simulink model "prob3"  (R2020b)
settings: Solver=VariableStepAuto  StartTime=0.0  StopTime=10.0  RelTol=1e-3
model workspace: external: MATLAB File C:\Users\deves\MATLAB\Projects\W2_problem3\data3.m (data not in the file)
values from neighbouring files (symbols this model uses):
  b = 50    [data3.m]
  M = 1000    [data3.m]
  U = 500    [data3.m]
settings Model: OrderedModelArguments=off  Creator=deves  LastModifiedBy=deves

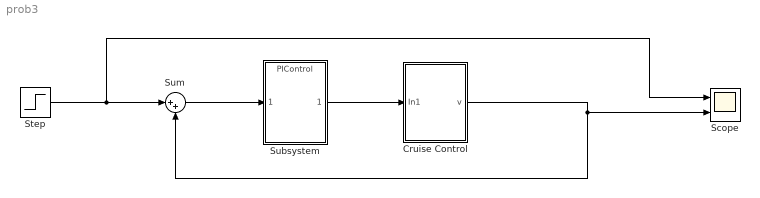
== system prob3 ==
  Cruise Control : Subsystem
  Scope : Scope  NumInputPorts=2
  Step : Step  After=U  SampleTime=0
  Subsystem : ModelReference  ModelNameDialog=PIControl  SimulationMode=Normal  ModelReferenceVersion=1.1
  Sum : Sum  Inputs=|++
  wires:
  Cruise Control/1(v) -> Sum/2, Scope/2
  Step/1 -> Scope/1, Sum/1
  Sum/1 -> Subsystem/1
  Subsystem/1 -> Cruise Control/1(In1)

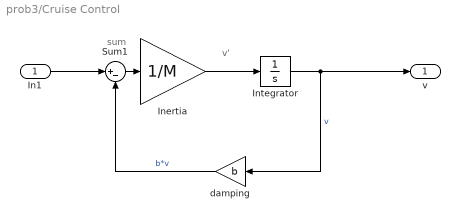
== system prob3/Cruise Control ==
  note: v'
  note: sum
  In1 : Inport
  Inertia : Gain  Gain=1/M
  Integrator : Integrator
  Sum1 : Sum  Inputs=|+-
  damping : Gain  Gain=b
  v : Outport
  wires:
  In1/1 -> Sum1/1
  damping/1 -> Sum1/2  "b*v"
  Integrator/1 -> v/1, damping/1  "v"
  Sum1/1 -> Inertia/1
  Inertia/1 -> Integrator/1
